simulink model "mdl5"  (Simulink 8.4)
settings: Solver=FixedStepDiscrete  SolverMode=SingleTasking  StartTime=TIME(1)  StopTime=TIME(end)  FixedStep=SIMSTEP  RelTol=1e-3
undefined symbols (not defined in the file): map_mr4_01, map_mr4_02, map_mr4_03, map_mr4_04, map_mr4_05, map_mr4_06, map_mr4_07, map_mr4_08, Parameter114, Parameter115, Parameter131, Parameter141, Parameter143, Parameter144, Parameter51, Parameter52, Parameter53, Parameter70, Parameter71, Parameter92, Parameter93, SIMSTEP
(part 2 of 3)

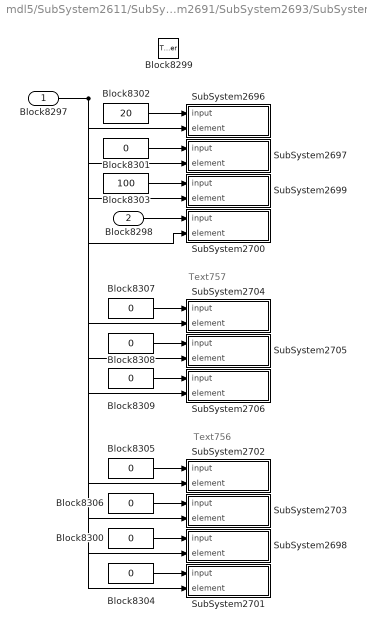
== system mdl5/SubSystem2611/SubSystem2691/SubSystem2693/SubSystem2695 ==
  note: Text757
  note: Text756
  Block8297 : Inport
  Block8298 : Inport  Port=2
  Block8299 : TriggerPort  TriggerType=function-call
  Block{8300..8301,8304..8309} (8 alike) : Constant  Value=0  OutDataTypeStr=double  SampleTime=-1
  Block8302 : Constant  Value=20  OutDataTypeStr=double  SampleTime=-1
  Block8303 : Constant  Value=100  OutDataTypeStr=double  SampleTime=-1
  SubSystem2696 : Subsystem  TreatAsAtomicUnit=on  mask(***ATC.DSWVEC***){bd_version=1.01.A, r0=DSM320, r1=-1, r2=, r3=, r4=, r5=, r6=, r7=, r8=, r9=, c0=, c1=, c2=, c3=, c4=, c5=, c6=, c7=, c8=, c9=}
      mask prompts: bd_version "Version"
      mask help: これはAutoCからのブロックです．編集禁止．
      settings: OpenFcn=warndlg('変更禁止!');
      mask Help: web(ui_blockhelpmng(gcb));
      mask Display: disp('ATC.DSRVEC')
  SubSystem2697 : Subsystem  TreatAsAtomicUnit=on  mask(***ATC.DSWVEC***){bd_version=1.01.A, r0=DSM319, r1=-1, r2=, r3=, r4=, r5=, r6=, r7=, r8=, r9=, c0=, c1=, c2=, c3=, c4=, c5=, c6=, c7=, c8=, c9=}
      mask prompts: bd_version "Version"
      mask help: これはAutoCからのブロックです．編集禁止．
      settings: OpenFcn=warndlg('変更禁止!');
      mask Help: web(ui_blockhelpmng(gcb));
      mask Display: disp('ATC.DSRVEC')
  SubSystem2698 : Subsystem  TreatAsAtomicUnit=on  mask(***ATC.DSWVEC***){bd_version=1.01.A, r0=DSM336, r1=-1, r2=, r3=, r4=, r5=, r6=, r7=, r8=, r9=, c0=, c1=, c2=, c3=, c4=, c5=, c6=, c7=, c8=, c9=}
      mask prompts: bd_version "Version"
      mask help: これはAutoCからのブロックです．編集禁止．
      settings: OpenFcn=warndlg('変更禁止!');
      mask Help: web(ui_blockhelpmng(gcb));
      mask Display: disp('ATC.DSRVEC')
  SubSystem2699 : Subsystem  TreatAsAtomicUnit=on  mask(***ATC.DSWVEC***){bd_version=1.01.A, r0=DSM318, r1=-1, r2=, r3=, r4=, r5=, r6=, r7=, r8=, r9=, c0=, c1=, c2=, c3=, c4=, c5=, c6=, c7=, c8=, c9=}
      mask prompts: bd_version "Version"
      mask help: これはAutoCからのブロックです．編集禁止．
      settings: OpenFcn=warndlg('変更禁止!');
      mask Help: web(ui_blockhelpmng(gcb));
      mask Display: disp('ATC.DSRVEC')
  SubSystem2700 : Subsystem  TreatAsAtomicUnit=on  mask(***ATC.DSWVEC***){bd_version=1.01.A, r0=DSM333, r1=-1, r2=, r3=, r4=, r5=, r6=, r7=, r8=, r9=, c0=, c1=, c2=, c3=, c4=, c5=, c6=, c7=, c8=, c9=}
      mask prompts: bd_version "Version"
      mask help: これはAutoCからのブロックです．編集禁止．
      settings: OpenFcn=warndlg('変更禁止!');
      mask Help: web(ui_blockhelpmng(gcb));
      mask Display: disp('ATC.DSRVEC')
  SubSystem2701 : Subsystem  TreatAsAtomicUnit=on  mask(***ATC.DSWVEC***){bd_version=1.01.A, r0=DSM337, r1=-1, r2=, r3=, r4=, r5=, r6=, r7=, r8=, r9=, c0=, c1=, c2=, c3=, c4=, c5=, c6=, c7=, c8=, c9=}
      mask prompts: bd_version "Version"
      mask help: これはAutoCからのブロックです．編集禁止．
      settings: OpenFcn=warndlg('変更禁止!');
      mask Help: web(ui_blockhelpmng(gcb));
      mask Display: disp('ATC.DSRVEC')
  SubSystem2702 : Subsystem  TreatAsAtomicUnit=on  mask(***ATC.DSWVEC***){bd_version=1.01.A, r0=DSM334, r1=-1, r2=, r3=, r4=, r5=, r6=, r7=, r8=, r9=, c0=, c1=, c2=, c3=, c4=, c5=, c6=, c7=, c8=, c9=}
      mask prompts: bd_version "Version"
      mask help: これはAutoCからのブロックです．編集禁止．
      settings: OpenFcn=warndlg('変更禁止!');
      mask Help: web(ui_blockhelpmng(gcb));
      mask Display: disp('ATC.DSRVEC')
  SubSystem2703 : Subsystem  TreatAsAtomicUnit=on  mask(***ATC.DSWVEC***){bd_version=1.01.A, r0=DSM335, r1=-1, r2=, r3=, r4=, r5=, r6=, r7=, r8=, r9=, c0=, c1=, c2=, c3=, c4=, c5=, c6=, c7=, c8=, c9=}
      mask prompts: bd_version "Version"
      mask help: これはAutoCからのブロックです．編集禁止．
      settings: OpenFcn=warndlg('変更禁止!');
      mask Help: web(ui_blockhelpmng(gcb));
      mask Display: disp('ATC.DSRVEC')
  SubSystem2704 : Subsystem  TreatAsAtomicUnit=on  mask(***ATC.DSWVEC***){bd_version=1.01.A, r0=DSM348, r1=-1, r2=, r3=, r4=, r5=, r6=, r7=, r8=, r9=, c0=, c1=, c2=, c3=, c4=, c5=, c6=, c7=, c8=, c9=}
      mask prompts: bd_version "Version"
      mask help: これはAutoCからのブロックです．編集禁止．
      settings: OpenFcn=warndlg('変更禁止!');
      mask Help: web(ui_blockhelpmng(gcb));
      mask Display: disp('ATC.DSRVEC')
  SubSystem2705 : Subsystem  TreatAsAtomicUnit=on  mask(***ATC.DSWVEC***){bd_version=1.01.A, r0=DSM349, r1=-1, r2=, r3=, r4=, r5=, r6=, r7=, r8=, r9=, c0=, c1=, c2=, c3=, c4=, c5=, c6=, c7=, c8=, c9=}
      mask prompts: bd_version "Version"
      mask help: これはAutoCからのブロックです．編集禁止．
      settings: OpenFcn=warndlg('変更禁止!');
      mask Help: web(ui_blockhelpmng(gcb));
      mask Display: disp('ATC.DSRVEC')
  SubSystem2706 : Subsystem  TreatAsAtomicUnit=on  mask(***ATC.DSWVEC***){bd_version=1.01.A, r0=DSM347, r1=-1, r2=, r3=, r4=, r5=, r6=, r7=, r8=, r9=, c0=, c1=, c2=, c3=, c4=, c5=, c6=, c7=, c8=, c9=}
      mask prompts: bd_version "Version"
      mask help: これはAutoCからのブロックです．編集禁止．
      settings: OpenFcn=warndlg('変更禁止!');
      mask Help: web(ui_blockhelpmng(gcb));
      mask Display: disp('ATC.DSRVEC')
  wires:
  Block8304/1 -> SubSystem2701/1(input)
  Block8305/1 -> SubSystem2702/1(input)
  Block8306/1 -> SubSystem2703/1(input)
  Block8300/1 -> SubSystem2698/1(input)
  Block8298/1 -> SubSystem2700/1(input)
  Block8302/1 -> SubSystem2696/1(input)
  Block8297/1 -> SubSystem2701/2(element), SubSystem2698/2(element), SubSystem2703/2(element), SubSystem2702/2(element), SubSystem2700/2(element), SubSystem2696/2(element), SubSystem2699/2(element), SubSystem2697/2(element), SubSystem2704/2(element), SubSystem2705/2(element), SubSystem2706/2(element)
  Block8301/1 -> SubSystem2697/1(input)
  Block8303/1 -> SubSystem2699/1(input)
  Block8307/1 -> SubSystem2704/1(input)
  Block8308/1 -> SubSystem2705/1(input)
  Block8309/1 -> SubSystem2706/1(input)

== system mdl5/SubSystem2611/SubSystem2612/SubSystem2620/SubSystem2624/SubSystem2625 ==
  note: ***編集禁止***
  input : Inport
  element : Inport  Port=2
  Assignment : Assignment  IndexOptions=Index vector (port)  OutputSizes=[1 1]
  Inside_DSR : DataStoreRead  DataStoreName=DSM319
  Inside_DSW : DataStoreWrite  DataStoreName=DSM319
  wires:
  element/1 -> Assignment/3
  input/1 -> Assignment/2
  Inside_DSR/1 -> Assignment/1
  Assignment/1 -> Inside_DSW/1

== system mdl5/SubSystem2611/SubSystem2612/SubSystem2620/SubSystem2624/SubSystem2626 ==
  note: ***編集禁止***
  input : Inport
  element : Inport  Port=2
  Assignment : Assignment  IndexOptions=Index vector (port)  OutputSizes=[1 1]
  Inside_DSR : DataStoreRead  DataStoreName=DSM333
  Inside_DSW : DataStoreWrite  DataStoreName=DSM333
  wires:
  element/1 -> Assignment/3
  input/1 -> Assignment/2
  Inside_DSR/1 -> Assignment/1
  Assignment/1 -> Inside_DSW/1

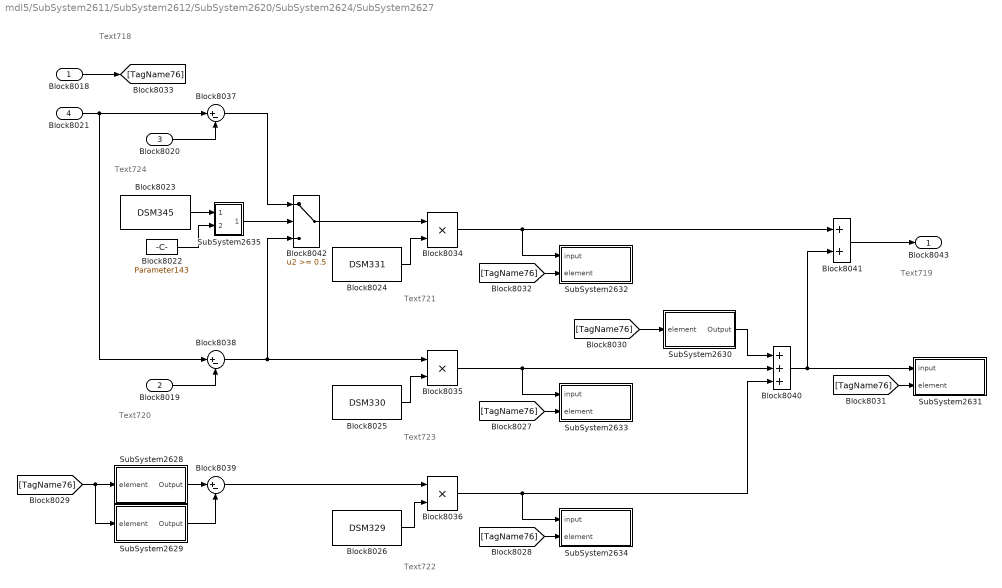
== system mdl5/SubSystem2611/SubSystem2612/SubSystem2620/SubSystem2624/SubSystem2627 ==
  note: Text724
  note: Text723
  note: Text722
  note: Text721
  note: Text720
  note: Text719
  note: Text718
  Block8018 : Inport
  Block8019 : Inport  Port=2
  Block8020 : Inport  Port=3
  Block8021 : Inport  Port=4
  Block8022 : Constant  Value=Parameter143  OutDataTypeStr=double  SampleTime=-1
  Block8023 : DataStoreRead  DataStoreName=DSM345
  Block8024 : DataStoreRead  DataStoreName=DSM331
  Block8025 : DataStoreRead  DataStoreName=DSM330
  Block8026 : DataStoreRead  DataStoreName=DSM329
  Block8034 : Product  OutDataTypeStr=double  SaturateOnIntegerOverflow=on  RndMeth=Zero  InputSameDT=on
  Block8035 : Product  OutDataTypeStr=double  SaturateOnIntegerOverflow=on  RndMeth=Zero  InputSameDT=on
  Block8036 : Product  OutDataTypeStr=double  SaturateOnIntegerOverflow=on  RndMeth=Zero  InputSameDT=on
  Block8037 : Sum  Inputs=|+-  OutDataTypeStr=double  RndMeth=Zero  SaturateOnIntegerOverflow=on  InputSameDT=on
  Block8038 : Sum  Inputs=|+-  OutDataTypeStr=double  RndMeth=Zero  SaturateOnIntegerOverflow=on  InputSameDT=on
  Block8039 : Sum  Inputs=|+-  OutDataTypeStr=double  RndMeth=Zero  SaturateOnIntegerOverflow=on  InputSameDT=on
  Block8040 : Sum  Inputs=+++  OutDataTypeStr=double  RndMeth=Zero  SaturateOnIntegerOverflow=on  InputSameDT=on
  Block8041 : Sum  OutDataTypeStr=double  RndMeth=Zero  SaturateOnIntegerOverflow=on  InputSameDT=on
  Block8042 : Switch  Threshold=0.5  RndMeth=Zero  SaturateOnIntegerOverflow=on  InputSameDT=on
  SubSystem2628 : Subsystem  TreatAsAtomicUnit=on  mask(***ATC.DSRVEC***){bd_version=1.01.A, r0=DSM147, r1=-1, r2=, r3=, r4=, r5=, r6=, r7=, r8=, r9=, c0=, c1=, c2=, c3=, c4=, c5=, c6=, c7=, c8=, c9=}
      mask prompts: bd_version "Version"
      mask help: これはAutoCからのブロックです．編集禁止．
      settings: OpenFcn=warndlg('変更禁止!');
      mask Help: web(ui_blockhelpmng(gcb));
      mask Display: disp('ATC.DSRVEC')
  SubSystem2629 : Subsystem  TreatAsAtomicUnit=on  mask(***ATC.DSRVEC***){bd_version=1.01.A, r0=DSM304, r1=-1, r2=, r3=, r4=, r5=, r6=, r7=, r8=, r9=, c0=, c1=, c2=, c3=, c4=, c5=, c6=, c7=, c8=, c9=}
      mask prompts: bd_version "Version"
      mask help: これはAutoCからのブロックです．編集禁止．
      settings: OpenFcn=warndlg('変更禁止!');
      mask Help: web(ui_blockhelpmng(gcb));
      mask Display: disp('ATC.DSRVEC')
  SubSystem2630 : Subsystem  Priority=1  TreatAsAtomicUnit=on  mask(***ATC.DSRVEC***){bd_version=1.01.A, r0=DSM346, r1=-1, r2=, r3=, r4=, r5=, r6=, r7=, r8=, r9=, c0=, c1=, c2=, c3=, c4=, c5=, c6=, c7=, c8=, c9=}
      mask prompts: bd_version "Version"
      mask help: これはAutoCからのブロックです．編集禁止．
      settings: AttributesFormatString=Attribute2091  OpenFcn=warndlg('変更禁止!');
      mask Help: web(ui_blockhelpmng(gcb));
      mask Display: disp('ATC.DSRVEC')
  SubSystem2631 : Subsystem  Priority=10  TreatAsAtomicUnit=on  mask(***ATC.DSWVEC***){bd_version=1.01.A, r0=DSM346, r1=-1, r2=, r3=, r4=, r5=, r6=, r7=, r8=, r9=, c0=, c1=, c2=, c3=, c4=, c5=, c6=, c7=, c8=, c9=}
      mask prompts: bd_version "Version"
      mask help: これはAutoCからのブロックです．編集禁止．
      settings: AttributesFormatString=Attribute2092  OpenFcn=warndlg('変更禁止!');
      mask Help: web(ui_blockhelpmng(gcb));
      mask Display: disp('ATC.DSRVEC')
  SubSystem2632 : Subsystem  TreatAsAtomicUnit=on  mask(***ATC.DSWVEC***){bd_version=1.01.A, r0=DSM349, r1=-1, r2=, r3=, r4=, r5=, r6=, r7=, r8=, r9=, c0=, c1=, c2=, c3=, c4=, c5=, c6=, c7=, c8=, c9=}
      mask prompts: bd_version "Version"
      mask help: これはAutoCからのブロックです．編集禁止．
      settings: OpenFcn=warndlg('変更禁止!');
      mask Help: web(ui_blockhelpmng(gcb));
      mask Display: disp('ATC.DSRVEC')
  SubSystem2633 : Subsystem  TreatAsAtomicUnit=on  mask(***ATC.DSWVEC***){bd_version=1.01.A, r0=DSM348, r1=-1, r2=, r3=, r4=, r5=, r6=, r7=, r8=, r9=, c0=, c1=, c2=, c3=, c4=, c5=, c6=, c7=, c8=, c9=}
      mask prompts: bd_version "Version"
      mask help: これはAutoCからのブロックです．編集禁止．
      settings: OpenFcn=warndlg('変更禁止!');
      mask Help: web(ui_blockhelpmng(gcb));
      mask Display: disp('ATC.DSRVEC')
  SubSystem2634 : Subsystem  TreatAsAtomicUnit=on  mask(***ATC.DSWVEC***){bd_version=1.01.A, r0=DSM347, r1=-1, r2=, r3=, r4=, r5=, r6=, r7=, r8=, r9=, c0=, c1=, c2=, c3=, c4=, c5=, c6=, c7=, c8=, c9=}
      mask prompts: bd_version "Version"
      mask help: これはAutoCからのブロックです．編集禁止．
      settings: OpenFcn=warndlg('変更禁止!');
      mask Help: web(ui_blockhelpmng(gcb));
      mask Display: disp('ATC.DSRVEC')
  SubSystem2635 : Subsystem
  Block8043 : Outport
  wires:
  [TagName76] -> SubSystem2629/1(element), SubSystem2628/1(element)
  SubSystem2629/1(Output) -> Block8039/2
  SubSystem2628/1(Output) -> Block8039/1
  Block8023/1 -> SubSystem2635/1(In1)
  Block8022/1 -> SubSystem2635/2(In2)
  Block8019/1 -> Block8038/2
  Block8020/1 -> Block8037/2
  Block8021/1 -> Block8037/1, Block8038/1
  SubSystem2635/1(Out1) -> Block8042/2
  Block8037/1 -> Block8042/1
  Block8038/1 -> Block8042/3, Block8035/1
  Block8042/1 -> Block8034/1
  Block8024/1 -> Block8034/2
  Block8025/1 -> Block8035/2
  Block8026/1 -> Block8036/2
  Block8039/1 -> Block8036/1
  Block8036/1 -> Block8040/3, SubSystem2634/1(input)
  Block8034/1 -> Block8041/1, SubSystem2632/1(input)
  Block8040/1 -> Block8041/2, SubSystem2631/1(input)
  [TagName76] -> SubSystem2630/1(element)
  Block8035/1 -> Block8040/2, SubSystem2633/1(input)
  SubSystem2630/1(Output) -> Block8040/1
  Block8041/1 -> Block8043/1
  [TagName76] -> SubSystem2631/2(element)
  [TagName76] -> SubSystem2632/2(element)
  [TagName76] -> SubSystem2633/2(element)
  [TagName76] -> SubSystem2634/2(element)
  Block8018/1 -> [TagName76]

== system mdl5/SubSystem2611/SubSystem2612/SubSystem2620/SubSystem2624/SubSystem2636 ==
  note: ***編集禁止***
  In1 : Inport
  In2 : Inport  Port=2
  RO1 : RelationalOperator  Operator===  InputSameDT=on
  single1 : DataTypeConversion  OutDataTypeStr=single  SaturateOnIntegerOverflow=on  RndMeth=Zero
  single2 : DataTypeConversion  OutDataTypeStr=single  SaturateOnIntegerOverflow=on  RndMeth=Zero
  Out1 : Outport
  wires:
  RO1/1 -> Out1/1
  In2/1 -> single2/1
  In1/1 -> single1/1
  single1/1 -> RO1/1
  single2/1 -> RO1/2

== system mdl5/SubSystem2611/SubSystem2612/SubSystem2620/SubSystem2624/SubSystem2637 ==
  note: ***編集禁止***
  Max : Inport
  Input : Inport  Port=2
  Min : Inport  Port=3
  Max1 : MinMax  Function=max  Inputs=2  SaturateOnIntegerOverflow=on  InputSameDT=on
  Min1 : MinMax  Inputs=2  SaturateOnIntegerOverflow=on  InputSameDT=on
  Output : Outport
  wires:
  Min1/1 -> Output/1
  Max/1 -> Min1/1
  Input/1 -> Max1/1
  Min/1 -> Max1/2
  Max1/1 -> Min1/2

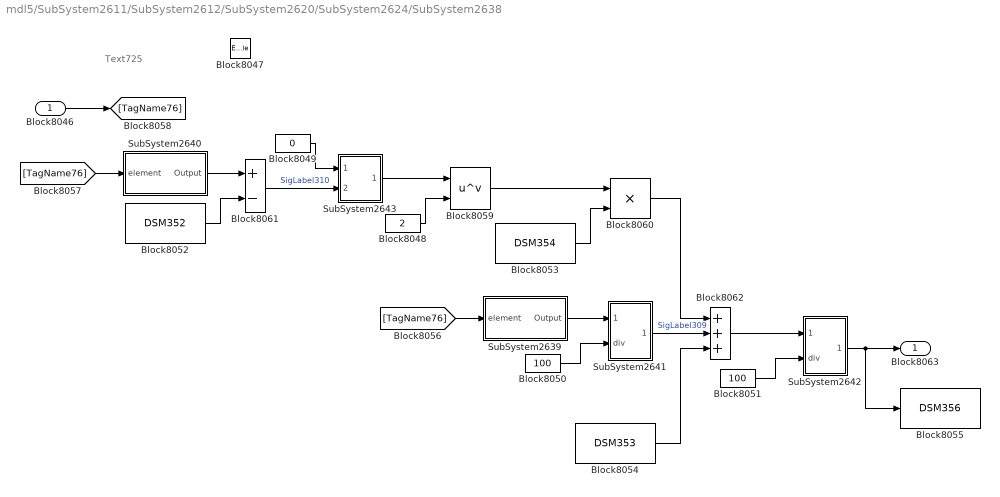
== system mdl5/SubSystem2611/SubSystem2612/SubSystem2620/SubSystem2624/SubSystem2638 ==
  note: Text725
  Block8046 : Inport
  Block8047 : EnablePort
  Block8048 : Constant  Value=2  OutDataTypeStr=double  SampleTime=-1
  Block8049 : Constant  Value=0  OutDataTypeStr=double  SampleTime=-1
  Block8050 : Constant  Value=100  OutDataTypeStr=double  SampleTime=-1
  Block8051 : Constant  Value=100  OutDataTypeStr=double  SampleTime=-1
  Block8052 : DataStoreRead  DataStoreName=DSM352
  Block8053 : DataStoreRead  DataStoreName=DSM354
  Block8054 : DataStoreRead  DataStoreName=DSM353
  Block8055 : DataStoreWrite  DataStoreName=DSM356
  Block8059 : Math  Operator=pow  SaturateOnIntegerOverflow=on
  Block8060 : Product  OutDataTypeStr=double  SaturateOnIntegerOverflow=on  RndMeth=Zero  InputSameDT=on
  Block8061 : Sum  Inputs=+-  OutDataTypeStr=double  RndMeth=Zero  SaturateOnIntegerOverflow=on  InputSameDT=on
  Block8062 : Sum  Inputs=+++  OutDataTypeStr=double  RndMeth=Zero  SaturateOnIntegerOverflow=on  InputSameDT=on
  SubSystem2639 : Subsystem  TreatAsAtomicUnit=on  mask(***ATC.DSRVEC***){bd_version=1.01.A, r0=DSM97, r1=-1, r2=, r3=, r4=, r5=, r6=, r7=, r8=, r9=, c0=, c1=, c2=, c3=, c4=, c5=, c6=, c7=, c8=, c9=}
      mask prompts: bd_version "Version"
      mask help: これはAutoCからのブロックです．編集禁止．
      settings: OpenFcn=warndlg('変更禁止!');
      mask Help: web(ui_blockhelpmng(gcb));
      mask Display: disp('ATC.DSRVEC')
  SubSystem2640 : Subsystem  TreatAsAtomicUnit=on  mask(***ATC.DSRVEC***){bd_version=1.01.A, r0=DSM318, r1=-1, r2=, r3=, r4=, r5=, r6=, r7=, r8=, r9=, c0=, c1=, c2=, c3=, c4=, c5=, c6=, c7=, c8=, c9=}
      mask prompts: bd_version "Version"
      mask help: これはAutoCからのブロックです．編集禁止．
      settings: OpenFcn=warndlg('変更禁止!');
      mask Help: web(ui_blockhelpmng(gcb));
      mask Display: disp('ATC.DSRVEC')
  SubSystem2641 : Subsystem  TreatAsAtomicUnit=on  mask(***ATC.DIVISION***){bd_version=1.01.A, r0=チェック無し, r1=, r2=, r3=, r4=, r5=, r6=, r7=, r8=, r9=, c0=, c1=, c2=, c3=, c4=, c5=, c6=, c7=, c8=, c9=}
      mask prompts: bd_version "Version"
      mask help: これはAutoCからのブロックです．編集禁止．
      settings: OpenFcn=warndlg('変更禁止!');
      mask Help: web(ui_blockhelpmng(gcb));
  SubSystem2642 : Subsystem  TreatAsAtomicUnit=on  mask(***ATC.DIVISION***){bd_version=1.01.A, r0=チェック無し, r1=, r2=, r3=, r4=, r5=, r6=, r7=, r8=, r9=, c0=, c1=, c2=, c3=, c4=, c5=, c6=, c7=, c8=, c9=}
      mask prompts: bd_version "Version"
      mask help: これはAutoCからのブロックです．編集禁止．
      settings: OpenFcn=warndlg('変更禁止!');
      mask Help: web(ui_blockhelpmng(gcb));
  SubSystem2643 : Subsystem  TreatAsAtomicUnit=on  mask(***ATC.SATURATION***){bd_version=1.01.A, r0=上限ガード, r1=上限ガード, r2=, r3=, r4=, r5=, r6=, r7=, r8=, r9=, c0=, c1=, c2=, c3=, c4=, c5=, c6=, c7=, c8=, c9=}
      mask prompts: bd_version "Version"
      mask help: これはAutoCからのブロックです．編集禁止．
      settings: OpenFcn=warndlg('変更禁止!');  RTWSystemCode=Inline
      mask Help: web(ui_blockhelpmng(gcb));
      mask Display:
      | plot([0 1],[0.3 0.3])
      | plot([0.5 0.5],[0 0.8])
      | plot([0.2 0.8],[0 0.7])
      | plot([0.8 1],[0.7 0.7])
      | plot([0 0],[1 1])
      | text(0.06,0.9,sprintf('Upper'))
  Block8063 : Outport
  wires:
  [TagName76] -> SubSystem2640/1(element)
  SubSystem2640/1(Output) -> Block8061/1
  Block8061/1 -> SubSystem2643/2(Input)  "SigLabel310"
  Block8049/1 -> SubSystem2643/1(Max)
  Block8053/1 -> Block8060/2
  Block8052/1 -> Block8061/2
  Block8054/1 -> Block8062/3
  Block8046/1 -> [TagName76]
  Block8059/1 -> Block8060/1
  SubSystem2643/1(Output) -> Block8059/1
  Block8048/1 -> Block8059/2
  SubSystem2639/1(Output) -> SubSystem2641/1(mult)
  Block8050/1 -> SubSystem2641/2(div)
  Block8060/1 -> Block8062/1
  SubSystem2641/1(Out) -> Block8062/2  "SigLabel309"
  [TagName76] -> SubSystem2639/1(element)
  Block8051/1 -> SubSystem2642/2(div)
  Block8062/1 -> SubSystem2642/1(mult)
  SubSystem2642/1(Out) -> Block8063/1, Block8055/1

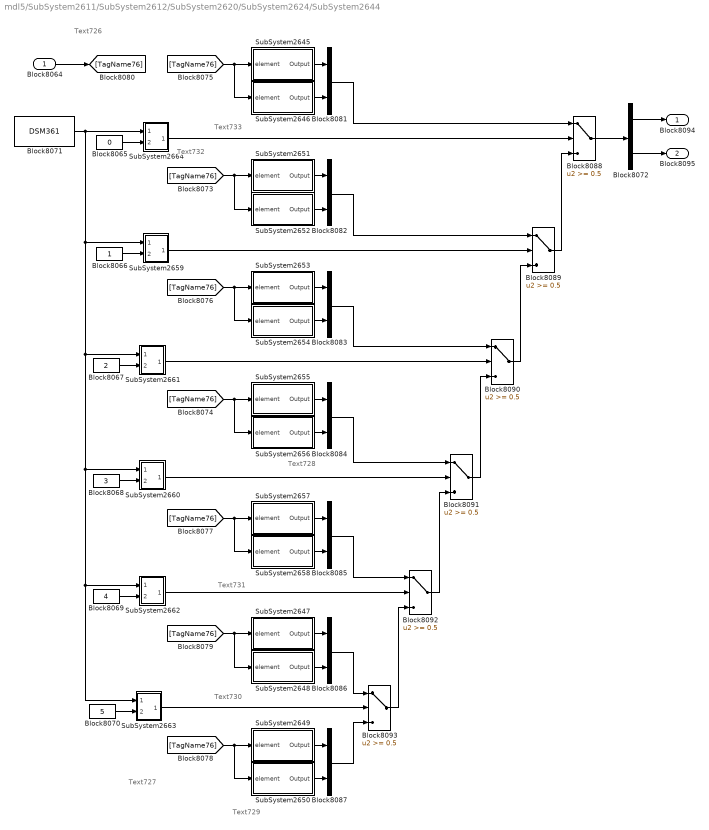
== system mdl5/SubSystem2611/SubSystem2612/SubSystem2620/SubSystem2624/SubSystem2644 ==
  note: Text733
  note: Text732
  note: Text731
  note: Text730
  note: Text729
  note: Text728
  note: Text727
  note: Text726
  Block8064 : Inport
  Block8065 : Constant  Value=0  OutDataTypeStr=double  SampleTime=-1
  Block8066 : Constant  OutDataTypeStr=double  SampleTime=-1
  Block8067 : Constant  Value=2  OutDataTypeStr=double  SampleTime=-1
  Block8068 : Constant  Value=3  OutDataTypeStr=double  SampleTime=-1
  Block8069 : Constant  Value=4  OutDataTypeStr=double  SampleTime=-1
  Block8070 : Constant  Value=5  OutDataTypeStr=double  SampleTime=-1
  Block8071 : DataStoreRead  DataStoreName=DSM361
  Block8072 : Demux  Outputs=2
  Block{8081..8087} (7 alike) : Mux  Inputs=2
  Block{8088..8093} (6 alike) : Switch  Threshold=0.5  RndMeth=Zero  SaturateOnIntegerOverflow=on  InputSameDT=on
  SubSystem2645 : Subsystem  TreatAsAtomicUnit=on  mask(***ATC.DSRVEC***){bd_version=1.01.A, r0=DSM115, r1=-1, r2=, r3=, r4=, r5=, r6=, r7=, r8=, r9=, c0=, c1=, c2=, c3=, c4=, c5=, c6=, c7=, c8=, c9=}
      mask prompts: bd_version "Version"
      mask help: これはAutoCからのブロックです．編集禁止．
      settings: OpenFcn=warndlg('変更禁止!');
      mask Help: web(ui_blockhelpmng(gcb));
      mask Display: disp('ATC.DSRVEC')
  SubSystem2646 : Subsystem  TreatAsAtomicUnit=on  mask(***ATC.DSRVEC***){bd_version=1.01.A, r0=DSM119, r1=-1, r2=, r3=, r4=, r5=, r6=, r7=, r8=, r9=, c0=, c1=, c2=, c3=, c4=, c5=, c6=, c7=, c8=, c9=}
      mask prompts: bd_version "Version"
      mask help: これはAutoCからのブロックです．編集禁止．
      settings: OpenFcn=warndlg('変更禁止!');
      mask Help: web(ui_blockhelpmng(gcb));
      mask Display: disp('ATC.DSRVEC')
  SubSystem2647 : Subsystem  TreatAsAtomicUnit=on  mask(***ATC.DSRVEC***){bd_version=1.01.A, r0=DSM102, r1=-1, r2=, r3=, r4=, r5=, r6=, r7=, r8=, r9=, c0=, c1=, c2=, c3=, c4=, c5=, c6=, c7=, c8=, c9=}
      mask prompts: bd_version "Version"
      mask help: これはAutoCからのブロックです．編集禁止．
      settings: OpenFcn=warndlg('変更禁止!');
      mask Help: web(ui_blockhelpmng(gcb));
      mask Display: disp('ATC.DSRVEC')
  SubSystem2648 : Subsystem  TreatAsAtomicUnit=on  mask(***ATC.DSRVEC***){bd_version=1.01.A, r0=DSM104, r1=-1, r2=, r3=, r4=, r5=, r6=, r7=, r8=, r9=, c0=, c1=, c2=, c3=, c4=, c5=, c6=, c7=, c8=, c9=}
      mask prompts: bd_version "Version"
      mask help: これはAutoCからのブロックです．編集禁止．
      settings: OpenFcn=warndlg('変更禁止!');
      mask Help: web(ui_blockhelpmng(gcb));
      mask Display: disp('ATC.DSRVEC')
  SubSystem2649 : Subsystem  TreatAsAtomicUnit=on  mask(***ATC.DSRVEC***){bd_version=1.01.A, r0=DSM110, r1=-1, r2=, r3=, r4=, r5=, r6=, r7=, r8=, r9=, c0=, c1=, c2=, c3=, c4=, c5=, c6=, c7=, c8=, c9=}
      mask prompts: bd_version "Version"
      mask help: これはAutoCからのブロックです．編集禁止．
      settings: OpenFcn=warndlg('変更禁止!');
      mask Help: web(ui_blockhelpmng(gcb));
      mask Display: disp('ATC.DSRVEC')
  SubSystem2650 : Subsystem  TreatAsAtomicUnit=on  mask(***ATC.DSRVEC***){bd_version=1.01.A, r0=DSM112, r1=-1, r2=, r3=, r4=, r5=, r6=, r7=, r8=, r9=, c0=, c1=, c2=, c3=, c4=, c5=, c6=, c7=, c8=, c9=}
      mask prompts: bd_version "Version"
      mask help: これはAutoCからのブロックです．編集禁止．
      settings: OpenFcn=warndlg('変更禁止!');
      mask Help: web(ui_blockhelpmng(gcb));
      mask Display: disp('ATC.DSRVEC')
  SubSystem2651 : Subsystem  TreatAsAtomicUnit=on  mask(***ATC.DSRVEC***){bd_version=1.01.A, r0=DSM116, r1=-1, r2=, r3=, r4=, r5=, r6=, r7=, r8=, r9=, c0=, c1=, c2=, c3=, c4=, c5=, c6=, c7=, c8=, c9=}
      mask prompts: bd_version "Version"
      mask help: これはAutoCからのブロックです．編集禁止．
      settings: OpenFcn=warndlg('変更禁止!');
      mask Help: web(ui_blockhelpmng(gcb));
      mask Display: disp('ATC.DSRVEC')
  SubSystem2652 : Subsystem  TreatAsAtomicUnit=on  mask(***ATC.DSRVEC***){bd_version=1.01.A, r0=DSM120, r1=-1, r2=, r3=, r4=, r5=, r6=, r7=, r8=, r9=, c0=, c1=, c2=, c3=, c4=, c5=, c6=, c7=, c8=, c9=}
      mask prompts: bd_version "Version"
      mask help: これはAutoCからのブロックです．編集禁止．
      settings: OpenFcn=warndlg('変更禁止!');
      mask Help: web(ui_blockhelpmng(gcb));
      mask Display: disp('ATC.DSRVEC')
  SubSystem2653 : Subsystem  TreatAsAtomicUnit=on  mask(***ATC.DSRVEC***){bd_version=1.01.A, r0=DSM122, r1=-1, r2=, r3=, r4=, r5=, r6=, r7=, r8=, r9=, c0=, c1=, c2=, c3=, c4=, c5=, c6=, c7=, c8=, c9=}
      mask prompts: bd_version "Version"
      mask help: これはAutoCからのブロックです．編集禁止．
      settings: OpenFcn=warndlg('変更禁止!');
      mask Help: web(ui_blockhelpmng(gcb));
      mask Display: disp('ATC.DSRVEC')
  SubSystem2654 : Subsystem  TreatAsAtomicUnit=on  mask(***ATC.DSRVEC***){bd_version=1.01.A, r0=DSM125, r1=-1, r2=, r3=, r4=, r5=, r6=, r7=, r8=, r9=, c0=, c1=, c2=, c3=, c4=, c5=, c6=, c7=, c8=, c9=}
      mask prompts: bd_version "Version"
      mask help: これはAutoCからのブロックです．編集禁止．
      settings: OpenFcn=warndlg('変更禁止!');
      mask Help: web(ui_blockhelpmng(gcb));
      mask Display: disp('ATC.DSRVEC')
  SubSystem2655 : Subsystem  TreatAsAtomicUnit=on  mask(***ATC.DSRVEC***){bd_version=1.01.A, r0=DSM123, r1=-1, r2=, r3=, r4=, r5=, r6=, r7=, r8=, r9=, c0=, c1=, c2=, c3=, c4=, c5=, c6=, c7=, c8=, c9=}
      mask prompts: bd_version "Version"
      mask help: これはAutoCからのブロックです．編集禁止．
      settings: OpenFcn=warndlg('変更禁止!');
      mask Help: web(ui_blockhelpmng(gcb));
      mask Display: disp('ATC.DSRVEC')
  SubSystem2656 : Subsystem  TreatAsAtomicUnit=on  mask(***ATC.DSRVEC***){bd_version=1.01.A, r0=DSM126, r1=-1, r2=, r3=, r4=, r5=, r6=, r7=, r8=, r9=, c0=, c1=, c2=, c3=, c4=, c5=, c6=, c7=, c8=, c9=}
      mask prompts: bd_version "Version"
      mask help: これはAutoCからのブロックです．編集禁止．
      settings: OpenFcn=warndlg('変更禁止!');
      mask Help: web(ui_blockhelpmng(gcb));
      mask Display: disp('ATC.DSRVEC')
  SubSystem2657 : Subsystem  TreatAsAtomicUnit=on  mask(***ATC.DSRVEC***){bd_version=1.01.A, r0=DSM106, r1=-1, r2=, r3=, r4=, r5=, r6=, r7=, r8=, r9=, c0=, c1=, c2=, c3=, c4=, c5=, c6=, c7=, c8=, c9=}
      mask prompts: bd_version "Version"
      mask help: これはAutoCからのブロックです．編集禁止．
      settings: OpenFcn=warndlg('変更禁止!');
      mask Help: web(ui_blockhelpmng(gcb));
      mask Display: disp('ATC.DSRVEC')
  SubSystem2658 : Subsystem  TreatAsAtomicUnit=on  mask(***ATC.DSRVEC***){bd_version=1.01.A, r0=DSM108, r1=-1, r2=, r3=, r4=, r5=, r6=, r7=, r8=, r9=, c0=, c1=, c2=, c3=, c4=, c5=, c6=, c7=, c8=, c9=}
      mask prompts: bd_version "Version"
      mask help: これはAutoCからのブロックです．編集禁止．
      settings: OpenFcn=warndlg('変更禁止!');
      mask Help: web(ui_blockhelpmng(gcb));
      mask Display: disp('ATC.DSRVEC')
  SubSystem2659 : Subsystem
  SubSystem2660 : Subsystem
  SubSystem2661 : Subsystem
  SubSystem2662 : Subsystem
  SubSystem2663 : Subsystem
  SubSystem2664 : Subsystem
  Block8094 : Outport
  Block8095 : Outport  Port=2
  wires:
  Block8064/1 -> [TagName76]
  SubSystem2645/1(Output) -> Block8081/1
  SubSystem2646/1(Output) -> Block8081/2
  [TagName76] -> SubSystem2645/1(element), SubSystem2646/1(element)
  Block8081/1 -> Block8088/1
  SubSystem2664/1(Out1) -> Block8088/2
  Block8065/1 -> SubSystem2664/2(In2)
  Block8071/1 -> SubSystem2664/1(In1), SubSystem2659/1(In1), SubSystem2661/1(In1), SubSystem2660/1(In1), SubSystem2662/1(In1), SubSystem2663/1(In1)
  SubSystem2651/1(Output) -> Block8082/1
  SubSystem2652/1(Output) -> Block8082/2
  [TagName76] -> SubSystem2652/1(element), SubSystem2651/1(element)
  Block8082/1 -> Block8089/1
  SubSystem2653/1(Output) -> Block8083/1
  SubSystem2654/1(Output) -> Block8083/2
  [TagName76] -> SubSystem2653/1(element), SubSystem2654/1(element)
  Block8083/1 -> Block8090/1
  SubSystem2655/1(Output) -> Block8084/1
  SubSystem2656/1(Output) -> Block8084/2
  [TagName76] -> SubSystem2656/1(element), SubSystem2655/1(element)
  Block8084/1 -> Block8091/1
  SubSystem2657/1(Output) -> Block8085/1
  SubSystem2658/1(Output) -> Block8085/2
  [TagName76] -> SubSystem2657/1(element), SubSystem2658/1(element)
  Block8085/1 -> Block8092/1
  SubSystem2647/1(Output) -> Block8086/1
  SubSystem2648/1(Output) -> Block8086/2
  [TagName76] -> SubSystem2648/1(element), SubSystem2647/1(element)
  Block8086/1 -> Block8093/1
  SubSystem2649/1(Output) -> Block8087/1
  SubSystem2650/1(Output) -> Block8087/2
  [TagName76] -> SubSystem2649/1(element), SubSystem2650/1(element)
  Block8066/1 -> SubSystem2659/2(In2)
  Block8068/1 -> SubSystem2660/2(In2)
  Block8069/1 -> SubSystem2662/2(In2)
  SubSystem2659/1(Out1) -> Block8089/2
  SubSystem2661/1(Out1) -> Block8090/2
  SubSystem2660/1(Out1) -> Block8091/2
  SubSystem2662/1(Out1) -> Block8092/2
  SubSystem2663/1(Out1) -> Block8093/2
  Block8087/1 -> Block8093/3
  Block8089/1 -> Block8088/3
  Block8090/1 -> Block8089/3
  Block8091/1 -> Block8090/3
  Block8092/1 -> Block8091/3
  Block8093/1 -> Block8092/3
  Block8067/1 -> SubSystem2661/2(In2)
  Block8070/1 -> SubSystem2663/2(In2)
  Block8088/1 -> Block8072/1
  Block8072/1 -> Block8094/1
  Block8072/2 -> Block8095/1

== system mdl5/SubSystem2611/SubSystem2612/SubSystem2665/SubSystem2666/SubSystem2667 ==
  note: ***編集禁止***
  input : Inport
  element : Inport  Port=2
  Assignment : Assignment  IndexOptions=Index vector (port)  OutputSizes=[1 1]
  Inside_DSR : DataStoreRead  DataStoreName=DSM320
  Inside_DSW : DataStoreWrite  DataStoreName=DSM320
  wires:
  Assignment/1 -> Inside_DSW/1
  Inside_DSR/1 -> Assignment/1
  input/1 -> Assignment/2
  element/1 -> Assignment/3

== system mdl5/SubSystem2611/SubSystem2612/SubSystem2665/SubSystem2666/SubSystem2668 ==
  note: ***編集禁止***
  In1 : Inport
  In2 : Inport  Port=2
  RO1 : RelationalOperator  Operator===  InputSameDT=on
  single1 : DataTypeConversion  OutDataTypeStr=single  SaturateOnIntegerOverflow=on  RndMeth=Zero
  single2 : DataTypeConversion  OutDataTypeStr=single  SaturateOnIntegerOverflow=on  RndMeth=Zero
  Out1 : Outport
  wires:
  RO1/1 -> Out1/1
  In2/1 -> single2/1
  In1/1 -> single1/1
  single1/1 -> RO1/1
  single2/1 -> RO1/2

== system mdl5/SubSystem2611/SubSystem2612/SubSystem2665/SubSystem2666/SubSystem2669 ==
  note: ***編集禁止***
  In1 : Inport
  In2 : Inport  Port=2
  RO1 : RelationalOperator  Operator===  InputSameDT=on
  single1 : DataTypeConversion  OutDataTypeStr=single  SaturateOnIntegerOverflow=on  RndMeth=Zero
  single2 : DataTypeConversion  OutDataTypeStr=single  SaturateOnIntegerOverflow=on  RndMeth=Zero
  Out1 : Outport
  wires:
  RO1/1 -> Out1/1
  In2/1 -> single2/1
  In1/1 -> single1/1
  single1/1 -> RO1/1
  single2/1 -> RO1/2

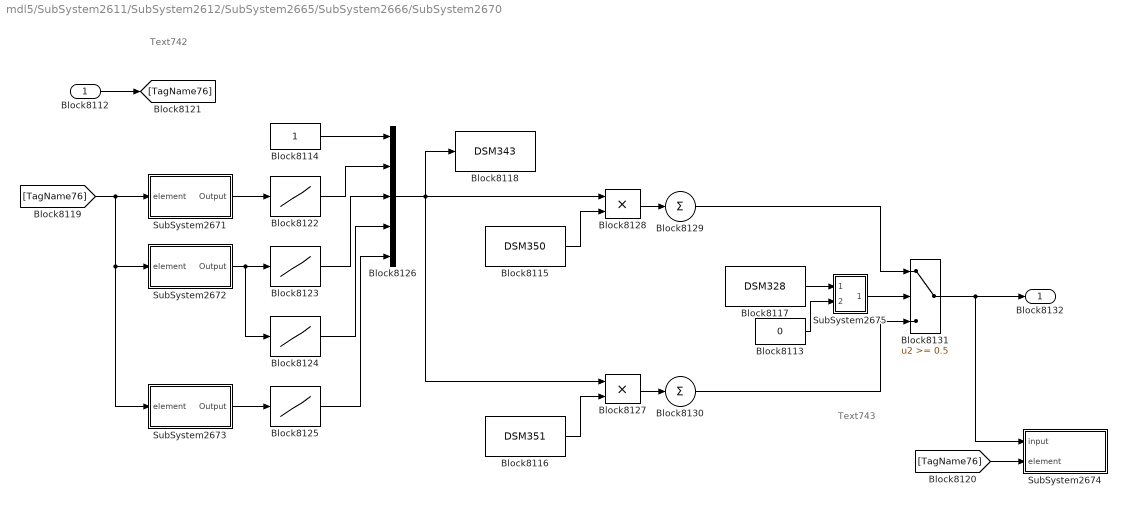
== system mdl5/SubSystem2611/SubSystem2612/SubSystem2665/SubSystem2666/SubSystem2670 ==
  note: Text743
  note: Text742
  Block8112 : Inport
  Block8113 : Constant  Value=0  OutDataTypeStr=double  SampleTime=-1
  Block8114 : Constant  OutDataTypeStr=double  SampleTime=-1
  Block8115 : DataStoreRead  DataStoreName=DSM350
  Block8116 : DataStoreRead  DataStoreName=DSM351
  Block8117 : DataStoreRead  DataStoreName=DSM328
  Block8118 : DataStoreWrite  DataStoreName=DSM343
  Block8122 : Lookup  InputValues=map_mr4_01  Table=map_mr4_02  SaturateOnIntegerOverflow=on
      settings: AttributesFormatString=<%<OutputValues>>\nAttribute2111
  Block8123 : Lookup  InputValues=map_mr4_03  Table=map_mr4_04  SaturateOnIntegerOverflow=on
      settings: AttributesFormatString=<%<OutputValues>>\nAttribute2112
  Block8124 : Lookup  InputValues=map_mr4_05  Table=map_mr4_06  SaturateOnIntegerOverflow=on
      settings: AttributesFormatString=<%<OutputValues>>\nAttribute2113
  Block8125 : Lookup  InputValues=map_mr4_07  Table=map_mr4_08  SaturateOnIntegerOverflow=on
      settings: AttributesFormatString=<%<OutputValues>>\nAttribute2114
  Block8126 : Mux  Inputs=5
  Block8127 : Product  OutDataTypeStr=double  SaturateOnIntegerOverflow=on  RndMeth=Zero  InputSameDT=on
  Block8128 : Product  OutDataTypeStr=double  SaturateOnIntegerOverflow=on  RndMeth=Zero  InputSameDT=on
  Block8129 : Sum  Inputs=+  OutDataTypeStr=double  RndMeth=Zero  SaturateOnIntegerOverflow=on  InputSameDT=on
  Block8130 : Sum  Inputs=+  OutDataTypeStr=double  RndMeth=Zero  SaturateOnIntegerOverflow=on  InputSameDT=on
  Block8131 : Switch  Threshold=0.5  RndMeth=Zero  SaturateOnIntegerOverflow=on  InputSameDT=on
  SubSystem2671 : Subsystem  TreatAsAtomicUnit=on  mask(***ATC.DSRVEC***){bd_version=1.01.A, r0=DSM97, r1=-1, r2=, r3=, r4=, r5=, r6=, r7=, r8=, r9=, c0=, c1=, c2=, c3=, c4=, c5=, c6=, c7=, c8=, c9=}
      mask prompts: bd_version "Version"
      mask help: これはAutoCからのブロックです．編集禁止．
      settings: OpenFcn=warndlg('変更禁止!');
      mask Help: web(ui_blockhelpmng(gcb));
      mask Display: disp('ATC.DSRVEC')
  SubSystem2672 : Subsystem  TreatAsAtomicUnit=on  mask(***ATC.DSRVEC***){bd_version=1.01.A, r0=DSM318, r1=-1, r2=, r3=, r4=, r5=, r6=, r7=, r8=, r9=, c0=, c1=, c2=, c3=, c4=, c5=, c6=, c7=, c8=, c9=}
      mask prompts: bd_version "Version"
      mask help: これはAutoCからのブロックです．編集禁止．
      settings: OpenFcn=warndlg('変更禁止!');
      mask Help: web(ui_blockhelpmng(gcb));
      mask Display: disp('ATC.DSRVEC')
  SubSystem2673 : Subsystem  TreatAsAtomicUnit=on  mask(***ATC.DSRVEC***){bd_version=1.01.A, r0=DSM36, r1=-1, r2=, r3=, r4=, r5=, r6=, r7=, r8=, r9=, c0=, c1=, c2=, c3=, c4=, c5=, c6=, c7=, c8=, c9=}
      mask prompts: bd_version "Version"
      mask help: これはAutoCからのブロックです．編集禁止．
      settings: OpenFcn=warndlg('変更禁止!');
      mask Help: web(ui_blockhelpmng(gcb));
      mask Display: disp('ATC.DSRVEC')
  SubSystem2674 : Subsystem  TreatAsAtomicUnit=on  mask(***ATC.DSWVEC***){bd_version=1.01.A, r0=DSM321, r1=-1, r2=, r3=, r4=, r5=, r6=, r7=, r8=, r9=, c0=, c1=, c2=, c3=, c4=, c5=, c6=, c7=, c8=, c9=}
      mask prompts: bd_version "Version"
      mask help: これはAutoCからのブロックです．編集禁止．
      settings: OpenFcn=warndlg('変更禁止!');
      mask Help: web(ui_blockhelpmng(gcb));
      mask Display: disp('ATC.DSRVEC')
  SubSystem2675 : Subsystem
  Block8132 : Outport
  wires:
  SubSystem2671/1(Output) -> Block8122/1
  SubSystem2672/1(Output) -> Block8124/1, Block8123/1
  SubSystem2673/1(Output) -> Block8125/1
  [TagName76] -> SubSystem2671/1(element), SubSystem2672/1(element), SubSystem2673/1(element)
  Block8126/1 -> Block8118/1, Block8128/1, Block8127/1
  Block8115/1 -> Block8128/2
  Block8116/1 -> Block8127/2
  Block8128/1 -> Block8129/1
  Block8131/1 -> Block8132/1, SubSystem2674/1(input)
  SubSystem2675/1(Out1) -> Block8131/2
  Block8117/1 -> SubSystem2675/1(In1)
  Block8113/1 -> SubSystem2675/2(In2)
  Block8127/1 -> Block8130/1
  Block8129/1 -> Block8131/1
  Block8114/1 -> Block8126/1
  Block8122/1 -> Block8126/2
  Block8123/1 -> Block8126/3
  Block8124/1 -> Block8126/4
  Block8125/1 -> Block8126/5
  [TagName76] -> SubSystem2674/2(element)
  Block8112/1 -> [TagName76]
  Block8130/1 -> Block8131/3

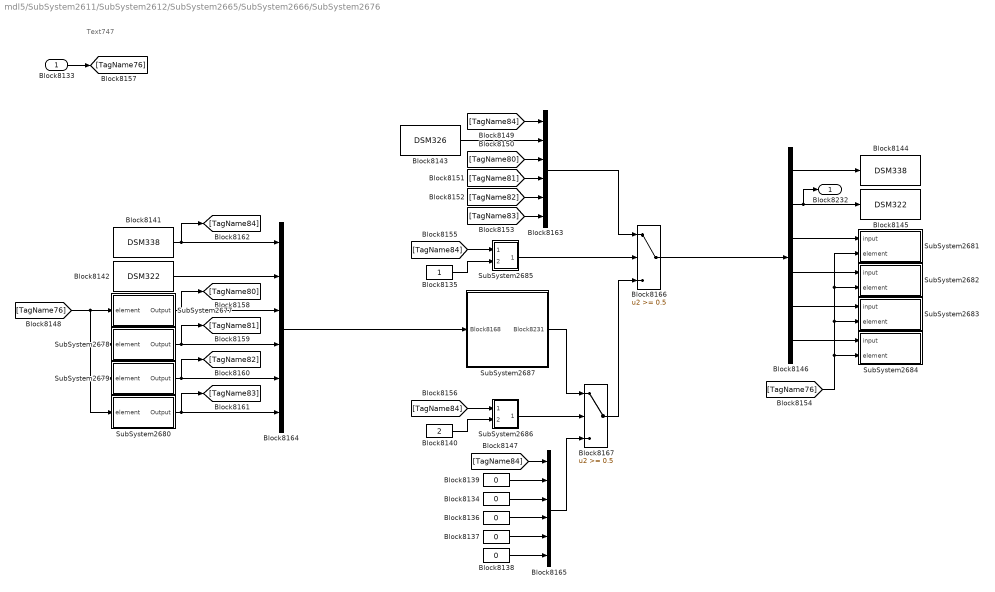
== system mdl5/SubSystem2611/SubSystem2612/SubSystem2665/SubSystem2666/SubSystem2676 ==
  note: Text747
  Block8133 : Inport
  Block{8134,8136..8139} (5 alike) : Constant  Value=0  OutDataTypeStr=double  SampleTime=-1
  Block8135 : Constant  OutDataTypeStr=double  SampleTime=-1
  Block8140 : Constant  Value=2  OutDataTypeStr=double  SampleTime=-1
  Block8141 : DataStoreRead  DataStoreName=DSM338
  Block8142 : DataStoreRead  DataStoreName=DSM322
  Block8143 : DataStoreRead  DataStoreName=DSM326
  Block8144 : DataStoreWrite  DataStoreName=DSM338
  Block8145 : DataStoreWrite  DataStoreName=DSM322
  Block8146 : Demux  Outputs=6
  Block8163 : Mux  Inputs=6
  Block8164 : Mux  Inputs=6
  Block8165 : Mux  Inputs=6
  Block8166 : Switch  Threshold=0.5  RndMeth=Zero  SaturateOnIntegerOverflow=on  InputSameDT=on
  Block8167 : Switch  Threshold=0.5  RndMeth=Zero  SaturateOnIntegerOverflow=on  InputSameDT=on
  SubSystem2677 : Subsystem  TreatAsAtomicUnit=on  mask(***ATC.DSRVEC***){bd_version=1.01.A, r0=DSM334, r1=-1, r2=, r3=, r4=, r5=, r6=, r7=, r8=, r9=, c0=, c1=, c2=, c3=, c4=, c5=, c6=, c7=, c8=, c9=}
      mask prompts: bd_version "Version"
      mask help: これはAutoCからのブロックです．編集禁止．
      settings: OpenFcn=warndlg('変更禁止!');
      mask Help: web(ui_blockhelpmng(gcb));
      mask Display: disp('ATC.DSRVEC')
  SubSystem2678 : Subsystem  TreatAsAtomicUnit=on  mask(***ATC.DSRVEC***){bd_version=1.01.A, r0=DSM335, r1=-1, r2=, r3=, r4=, r5=, r6=, r7=, r8=, r9=, c0=, c1=, c2=, c3=, c4=, c5=, c6=, c7=, c8=, c9=}
      mask prompts: bd_version "Version"
      mask help: これはAutoCからのブロックです．編集禁止．
      settings: OpenFcn=warndlg('変更禁止!');
      mask Help: web(ui_blockhelpmng(gcb));
      mask Display: disp('ATC.DSRVEC')
  SubSystem2679 : Subsystem  TreatAsAtomicUnit=on  mask(***ATC.DSRVEC***){bd_version=1.01.A, r0=DSM336, r1=-1, r2=, r3=, r4=, r5=, r6=, r7=, r8=, r9=, c0=, c1=, c2=, c3=, c4=, c5=, c6=, c7=, c8=, c9=}
      mask prompts: bd_version "Version"
      mask help: これはAutoCからのブロックです．編集禁止．
      settings: OpenFcn=warndlg('変更禁止!');
      mask Help: web(ui_blockhelpmng(gcb));
      mask Display: disp('ATC.DSRVEC')
  SubSystem2680 : Subsystem  TreatAsAtomicUnit=on  mask(***ATC.DSRVEC***){bd_version=1.01.A, r0=DSM337, r1=-1, r2=, r3=, r4=, r5=, r6=, r7=, r8=, r9=, c0=, c1=, c2=, c3=, c4=, c5=, c6=, c7=, c8=, c9=}
      mask prompts: bd_version "Version"
      mask help: これはAutoCからのブロックです．編集禁止．
      settings: OpenFcn=warndlg('変更禁止!');
      mask Help: web(ui_blockhelpmng(gcb));
      mask Display: disp('ATC.DSRVEC')
  SubSystem2681 : Subsystem  TreatAsAtomicUnit=on  mask(***ATC.DSWVEC***){bd_version=1.01.A, r0=DSM334, r1=-1, r2=, r3=, r4=, r5=, r6=, r7=, r8=, r9=, c0=, c1=, c2=, c3=, c4=, c5=, c6=, c7=, c8=, c9=}
      mask prompts: bd_version "Version"
      mask help: これはAutoCからのブロックです．編集禁止．
      settings: OpenFcn=warndlg('変更禁止!');
      mask Help: web(ui_blockhelpmng(gcb));
      mask Display: disp('ATC.DSRVEC')
  SubSystem2682 : Subsystem  TreatAsAtomicUnit=on  mask(***ATC.DSWVEC***){bd_version=1.01.A, r0=DSM335, r1=-1, r2=, r3=, r4=, r5=, r6=, r7=, r8=, r9=, c0=, c1=, c2=, c3=, c4=, c5=, c6=, c7=, c8=, c9=}
      mask prompts: bd_version "Version"
      mask help: これはAutoCからのブロックです．編集禁止．
      settings: OpenFcn=warndlg('変更禁止!');
      mask Help: web(ui_blockhelpmng(gcb));
      mask Display: disp('ATC.DSRVEC')
  SubSystem2683 : Subsystem  TreatAsAtomicUnit=on  mask(***ATC.DSWVEC***){bd_version=1.01.A, r0=DSM336, r1=-1, r2=, r3=, r4=, r5=, r6=, r7=, r8=, r9=, c0=, c1=, c2=, c3=, c4=, c5=, c6=, c7=, c8=, c9=}
      mask prompts: bd_version "Version"
      mask help: これはAutoCからのブロックです．編集禁止．
      settings: OpenFcn=warndlg('変更禁止!');
      mask Help: web(ui_blockhelpmng(gcb));
      mask Display: disp('ATC.DSRVEC')
  SubSystem2684 : Subsystem  TreatAsAtomicUnit=on  mask(***ATC.DSWVEC***){bd_version=1.01.A, r0=DSM337, r1=-1, r2=, r3=, r4=, r5=, r6=, r7=, r8=, r9=, c0=, c1=, c2=, c3=, c4=, c5=, c6=, c7=, c8=, c9=}
      mask prompts: bd_version "Version"
      mask help: これはAutoCからのブロックです．編集禁止．
      settings: OpenFcn=warndlg('変更禁止!');
      mask Help: web(ui_blockhelpmng(gcb));
      mask Display: disp('ATC.DSRVEC')
  SubSystem2685 : Subsystem
  SubSystem2686 : Subsystem
  SubSystem2687 : Subsystem  TreatAsAtomicUnit=on
  Block8232 : Outport
  wires:
  [TagName76] -> SubSystem2681/2(element), SubSystem2682/2(element), SubSystem2683/2(element), SubSystem2684/2(element)
  SubSystem2687/1(Block8231) -> Block8167/1
  Block8133/1 -> [TagName76]
  Block8164/1 -> SubSystem2687/1(Block8168)
  Block8141/1 -> [TagName84], Block8164/1
  Block8142/1 -> Block8164/2
  SubSystem2677/1(Output) -> [TagName80], Block8164/3
  SubSystem2678/1(Output) -> [TagName81], Block8164/4
  SubSystem2679/1(Output) -> [TagName82], Block8164/5
  SubSystem2680/1(Output) -> [TagName83], Block8164/6
  [TagName84] -> SubSystem2685/1(In1)
  Block8135/1 -> SubSystem2685/2(In2)
  [TagName84] -> SubSystem2686/1(In1)
  Block8140/1 -> SubSystem2686/2(In2)
  SubSystem2685/1(Out1) -> Block8166/2
  SubSystem2686/1(Out1) -> Block8167/2
  Block8163/1 -> Block8166/1
  Block8165/1 -> Block8167/3
  [TagName76] -> SubSystem2677/1(element), SubSystem2678/1(element), SubSystem2679/1(element), SubSystem2680/1(element)
  Block8166/1 -> Block8146/1
  Block8167/1 -> Block8166/3
  Block8146/1 -> Block8144/1
  Block8146/2 -> Block8145/1, Block8232/1
  Block8146/3 -> SubSystem2681/1(input)
  Block8146/4 -> SubSystem2682/1(input)
  Block8146/5 -> SubSystem2683/1(input)
  Block8146/6 -> SubSystem2684/1(input)
  [TagName84] -> Block8163/1
  Block8143/1 -> Block8163/2
  [TagName80] -> Block8163/3
  [TagName81] -> Block8163/4
  [TagName82] -> Block8163/5
  [TagName83] -> Block8163/6
  [TagName84] -> Block8165/1
  Block8139/1 -> Block8165/2
  Block8134/1 -> Block8165/3
  Block8136/1 -> Block8165/4
  Block8137/1 -> Block8165/5
  Block8138/1 -> Block8165/6

== system mdl5/SubSystem2611/SubSystem2691/SubSystem2693/SubSystem2695/SubSystem2696 ==
  note: ***編集禁止***
  input : Inport
  element : Inport  Port=2
  Assignment : Assignment  IndexOptions=Index vector (port)  OutputSizes=[1 1]
  Inside_DSR : DataStoreRead  DataStoreName=DSM320
  Inside_DSW : DataStoreWrite  DataStoreName=DSM320
  wires:
  Assignment/1 -> Inside_DSW/1
  Inside_DSR/1 -> Assignment/1
  input/1 -> Assignment/2
  element/1 -> Assignment/3

== system mdl5/SubSystem2611/SubSystem2691/SubSystem2693/SubSystem2695/SubSystem2697 ==
  note: ***編集禁止***
  input : Inport
  element : Inport  Port=2
  Assignment : Assignment  IndexOptions=Index vector (port)  OutputSizes=[1 1]
  Inside_DSR : DataStoreRead  DataStoreName=DSM319
  Inside_DSW : DataStoreWrite  DataStoreName=DSM319
  wires:
  Assignment/1 -> Inside_DSW/1
  Inside_DSR/1 -> Assignment/1
  input/1 -> Assignment/2
  element/1 -> Assignment/3

== system mdl5/SubSystem2611/SubSystem2691/SubSystem2693/SubSystem2695/SubSystem2698 ==
  note: ***編集禁止***
  input : Inport
  element : Inport  Port=2
  Assignment : Assignment  IndexOptions=Index vector (port)  OutputSizes=[1 1]
  Inside_DSR : DataStoreRead  DataStoreName=DSM336
  Inside_DSW : DataStoreWrite  DataStoreName=DSM336
  wires:
  element/1 -> Assignment/3
  input/1 -> Assignment/2
  Inside_DSR/1 -> Assignment/1
  Assignment/1 -> Inside_DSW/1

== system mdl5/SubSystem2611/SubSystem2691/SubSystem2693/SubSystem2695/SubSystem2699 ==
  note: ***編集禁止***
  input : Inport
  element : Inport  Port=2
  Assignment : Assignment  IndexOptions=Index vector (port)  OutputSizes=[1 1]
  Inside_DSR : DataStoreRead  DataStoreName=DSM318
  Inside_DSW : DataStoreWrite  DataStoreName=DSM318
  wires:
  Assignment/1 -> Inside_DSW/1
  Inside_DSR/1 -> Assignment/1
  input/1 -> Assignment/2
  element/1 -> Assignment/3

== system mdl5/SubSystem2611/SubSystem2691/SubSystem2693/SubSystem2695/SubSystem2700 ==
  note: ***編集禁止***
  input : Inport
  element : Inport  Port=2
  Assignment : Assignment  IndexOptions=Index vector (port)  OutputSizes=[1 1]
  Inside_DSR : DataStoreRead  DataStoreName=DSM333
  Inside_DSW : DataStoreWrite  DataStoreName=DSM333
  wires:
  element/1 -> Assignment/3
  input/1 -> Assignment/2
  Inside_DSR/1 -> Assignment/1
  Assignment/1 -> Inside_DSW/1

== system mdl5/SubSystem2611/SubSystem2691/SubSystem2693/SubSystem2695/SubSystem2701 ==
  note: ***編集禁止***
  input : Inport
  element : Inport  Port=2
  Assignment : Assignment  IndexOptions=Index vector (port)  OutputSizes=[1 1]
  Inside_DSR : DataStoreRead  DataStoreName=DSM337
  Inside_DSW : DataStoreWrite  DataStoreName=DSM337
  wires:
  Assignment/1 -> Inside_DSW/1
  Inside_DSR/1 -> Assignment/1
  input/1 -> Assignment/2
  element/1 -> Assignment/3

== system mdl5/SubSystem2611/SubSystem2691/SubSystem2693/SubSystem2695/SubSystem2702 ==
  note: ***編集禁止***
  input : Inport
  element : Inport  Port=2
  Assignment : Assignment  IndexOptions=Index vector (port)  OutputSizes=[1 1]
  Inside_DSR : DataStoreRead  DataStoreName=DSM334
  Inside_DSW : DataStoreWrite  DataStoreName=DSM334
  wires:
  element/1 -> Assignment/3
  input/1 -> Assignment/2
  Inside_DSR/1 -> Assignment/1
  Assignment/1 -> Inside_DSW/1

== system mdl5/SubSystem2611/SubSystem2691/SubSystem2693/SubSystem2695/SubSystem2703 ==
  note: ***編集禁止***
  input : Inport
  element : Inport  Port=2
  Assignment : Assignment  IndexOptions=Index vector (port)  OutputSizes=[1 1]
  Inside_DSR : DataStoreRead  DataStoreName=DSM335
  Inside_DSW : DataStoreWrite  DataStoreName=DSM335
  wires:
  element/1 -> Assignment/3
  input/1 -> Assignment/2
  Inside_DSR/1 -> Assignment/1
  Assignment/1 -> Inside_DSW/1

== system mdl5/SubSystem2611/SubSystem2691/SubSystem2693/SubSystem2695/SubSystem2704 ==
  note: ***編集禁止***
  input : Inport
  element : Inport  Port=2
  Assignment : Assignment  IndexOptions=Index vector (port)  OutputSizes=[1 1]
  Inside_DSR : DataStoreRead  DataStoreName=DSM348
  Inside_DSW : DataStoreWrite  DataStoreName=DSM348
  wires:
  Assignment/1 -> Inside_DSW/1
  Inside_DSR/1 -> Assignment/1
  input/1 -> Assignment/2
  element/1 -> Assignment/3

== system mdl5/SubSystem2611/SubSystem2691/SubSystem2693/SubSystem2695/SubSystem2705 ==
  note: ***編集禁止***
  input : Inport
  element : Inport  Port=2
  Assignment : Assignment  IndexOptions=Index vector (port)  OutputSizes=[1 1]
  Inside_DSR : DataStoreRead  DataStoreName=DSM349
  Inside_DSW : DataStoreWrite  DataStoreName=DSM349
  wires:
  Assignment/1 -> Inside_DSW/1
  Inside_DSR/1 -> Assignment/1
  input/1 -> Assignment/2
  element/1 -> Assignment/3

== system mdl5/SubSystem2611/SubSystem2691/SubSystem2693/SubSystem2695/SubSystem2706 ==
  note: ***編集禁止***
  input : Inport
  element : Inport  Port=2
  Assignment : Assignment  IndexOptions=Index vector (port)  OutputSizes=[1 1]
  Inside_DSR : DataStoreRead  DataStoreName=DSM347
  Inside_DSW : DataStoreWrite  DataStoreName=DSM347
  wires:
  Assignment/1 -> Inside_DSW/1
  Inside_DSR/1 -> Assignment/1
  input/1 -> Assignment/2
  element/1 -> Assignment/3

== system mdl5/SubSystem2611/SubSystem2612/SubSystem2620/SubSystem2624/SubSystem2627/SubSystem2628 ==
  note: ***編集禁止***
  element : Inport
  Inside_DSR : DataStoreRead  DataStoreName=DSM147
  Selector : Selector  IndexOptions=Index vector (port)  Indices=[1 3]
  Output : Outport
  wires:
  Selector/1 -> Output/1
  element/1 -> Selector/2
  Inside_DSR/1 -> Selector/1

== system mdl5/SubSystem2611/SubSystem2612/SubSystem2620/SubSystem2624/SubSystem2627/SubSystem2629 ==
  note: ***編集禁止***
  element : Inport
  Inside_DSR : DataStoreRead  DataStoreName=DSM304
  Selector : Selector  IndexOptions=Index vector (port)  Indices=[1 3]
  Output : Outport
  wires:
  Inside_DSR/1 -> Selector/1
  element/1 -> Selector/2
  Selector/1 -> Output/1

== system mdl5/SubSystem2611/SubSystem2612/SubSystem2620/SubSystem2624/SubSystem2627/SubSystem2630 ==
  note: ***編集禁止***
  element : Inport
  Inside_DSR : DataStoreRead  DataStoreName=DSM346
  Selector : Selector  IndexOptions=Index vector (port)  Indices=[1 3]
  Output : Outport
  wires:
  Selector/1 -> Output/1
  element/1 -> Selector/2
  Inside_DSR/1 -> Selector/1

== system mdl5/SubSystem2611/SubSystem2612/SubSystem2620/SubSystem2624/SubSystem2627/SubSystem2631 ==
  note: ***編集禁止***
  input : Inport
  element : Inport  Port=2
  Assignment : Assignment  IndexOptions=Index vector (port)  OutputSizes=[1 1]
  Inside_DSR : DataStoreRead  DataStoreName=DSM346
  Inside_DSW : DataStoreWrite  DataStoreName=DSM346
  wires:
  Assignment/1 -> Inside_DSW/1
  Inside_DSR/1 -> Assignment/1
  input/1 -> Assignment/2
  element/1 -> Assignment/3

== system mdl5/SubSystem2611/SubSystem2612/SubSystem2620/SubSystem2624/SubSystem2627/SubSystem2632 ==
  note: ***編集禁止***
  input : Inport
  element : Inport  Port=2
  Assignment : Assignment  IndexOptions=Index vector (port)  OutputSizes=[1 1]
  Inside_DSR : DataStoreRead  DataStoreName=DSM349
  Inside_DSW : DataStoreWrite  DataStoreName=DSM349
  wires:
  Assignment/1 -> Inside_DSW/1
  Inside_DSR/1 -> Assignment/1
  input/1 -> Assignment/2
  element/1 -> Assignment/3

== system mdl5/SubSystem2611/SubSystem2612/SubSystem2620/SubSystem2624/SubSystem2627/SubSystem2633 ==
  note: ***編集禁止***
  input : Inport
  element : Inport  Port=2
  Assignment : Assignment  IndexOptions=Index vector (port)  OutputSizes=[1 1]
  Inside_DSR : DataStoreRead  DataStoreName=DSM348
  Inside_DSW : DataStoreWrite  DataStoreName=DSM348
  wires:
  element/1 -> Assignment/3
  input/1 -> Assignment/2
  Inside_DSR/1 -> Assignment/1
  Assignment/1 -> Inside_DSW/1

== system mdl5/SubSystem2611/SubSystem2612/SubSystem2620/SubSystem2624/SubSystem2627/SubSystem2634 ==
  note: ***編集禁止***
  input : Inport
  element : Inport  Port=2
  Assignment : Assignment  IndexOptions=Index vector (port)  OutputSizes=[1 1]
  Inside_DSR : DataStoreRead  DataStoreName=DSM347
  Inside_DSW : DataStoreWrite  DataStoreName=DSM347
  wires:
  element/1 -> Assignment/3
  input/1 -> Assignment/2
  Inside_DSR/1 -> Assignment/1
  Assignment/1 -> Inside_DSW/1

== system mdl5/SubSystem2611/SubSystem2612/SubSystem2620/SubSystem2624/SubSystem2627/SubSystem2635 ==
  note: ***編集禁止***
  In1 : Inport
  In2 : Inport  Port=2
  RO1 : RelationalOperator  Operator===  InputSameDT=on
  single1 : DataTypeConversion  OutDataTypeStr=single  SaturateOnIntegerOverflow=on  RndMeth=Zero
  single2 : DataTypeConversion  OutDataTypeStr=single  SaturateOnIntegerOverflow=on  RndMeth=Zero
  Out1 : Outport
  wires:
  single2/1 -> RO1/2
  single1/1 -> RO1/1
  In1/1 -> single1/1
  In2/1 -> single2/1
  RO1/1 -> Out1/1

== system mdl5/SubSystem2611/SubSystem2612/SubSystem2620/SubSystem2624/SubSystem2638/SubSystem2639 ==
  note: ***編集禁止***
  element : Inport
  Inside_DSR : DataStoreRead  DataStoreName=DSM97
  Selector : Selector  IndexOptions=Index vector (port)  Indices=[1 3]
  Output : Outport
  wires:
  Inside_DSR/1 -> Selector/1
  element/1 -> Selector/2
  Selector/1 -> Output/1

== system mdl5/SubSystem2611/SubSystem2612/SubSystem2620/SubSystem2624/SubSystem2638/SubSystem2640 ==
  note: ***編集禁止***
  element : Inport
  Inside_DSR : DataStoreRead  DataStoreName=DSM318
  Selector : Selector  IndexOptions=Index vector (port)  Indices=[1 3]
  Output : Outport
  wires:
  Selector/1 -> Output/1
  element/1 -> Selector/2
  Inside_DSR/1 -> Selector/1

== system mdl5/SubSystem2611/SubSystem2612/SubSystem2620/SubSystem2624/SubSystem2638/SubSystem2641 ==
  note: ***編集禁止***
  mult : Inport
  div : Inport  Port=2
  Product : Product  Inputs=*/  SaturateOnIntegerOverflow=on  RndMeth=Zero  InputSameDT=on  OutDataTypeStr=Inherit: Same as first input
  Out : Outport
  wires:
  div/1 -> Product/2
  mult/1 -> Product/1
  Product/1 -> Out/1

== system mdl5/SubSystem2611/SubSystem2612/SubSystem2620/SubSystem2624/SubSystem2638/SubSystem2642 ==
  note: ***編集禁止***
  mult : Inport
  div : Inport  Port=2
  Product : Product  Inputs=*/  SaturateOnIntegerOverflow=on  RndMeth=Zero  InputSameDT=on  OutDataTypeStr=Inherit: Same as first input
  Out : Outport
  wires:
  Product/1 -> Out/1
  mult/1 -> Product/1
  div/1 -> Product/2

== system mdl5/SubSystem2611/SubSystem2612/SubSystem2620/SubSystem2624/SubSystem2638/SubSystem2643 ==
  note: ***編集禁止***
  Max : Inport
  Input : Inport  Port=2
  Min1 : MinMax  Inputs=2  SaturateOnIntegerOverflow=on  InputSameDT=on
  Output : Outport
  wires:
  Max/1 -> Min1/1
  Input/1 -> Min1/2
  Min1/1 -> Output/1

== system mdl5/SubSystem2611/SubSystem2612/SubSystem2620/SubSystem2624/SubSystem2644/SubSystem2645 ==
  note: ***編集禁止***
  element : Inport
  Inside_DSR : DataStoreRead  DataStoreName=DSM115
  Selector : Selector  IndexOptions=Index vector (port)  Indices=[1 3]
  Output : Outport
  wires:
  Inside_DSR/1 -> Selector/1
  element/1 -> Selector/2
  Selector/1 -> Output/1

== system mdl5/SubSystem2611/SubSystem2612/SubSystem2620/SubSystem2624/SubSystem2644/SubSystem2646 ==
  note: ***編集禁止***
  element : Inport
  Inside_DSR : DataStoreRead  DataStoreName=DSM119
  Selector : Selector  IndexOptions=Index vector (port)  Indices=[1 3]
  Output : Outport
  wires:
  Selector/1 -> Output/1
  element/1 -> Selector/2
  Inside_DSR/1 -> Selector/1

== system mdl5/SubSystem2611/SubSystem2612/SubSystem2620/SubSystem2624/SubSystem2644/SubSystem2647 ==
  note: ***編集禁止***
  element : Inport
  Inside_DSR : DataStoreRead  DataStoreName=DSM102
  Selector : Selector  IndexOptions=Index vector (port)  Indices=[1 3]
  Output : Outport
  wires:
  Selector/1 -> Output/1
  element/1 -> Selector/2
  Inside_DSR/1 -> Selector/1
